simulink model "TCC"  (R2022b)
settings: configuration reference "ERT" (kept outside this file)
undefined symbols (not defined in the file): DFC, ECM, EGM, facTrqDmpGain_C, facTrqRateLim_C, FID, kiMultdtNCtrl_C, kiMultdtPosnCtrl_C, kpNCtrl_C, kpPosnCtrl_C, SpdSetAlOfsCal_C, tauTrqDmpAvrg_C, tauTrqDmpDelay_C, tiPosnHold_C, trqPMaxNCtrl_C, trqPMaxPosnCtrl_C, TrqSetAlOfsCal_C
libraries: simulink x7, DSMLib x2, MathLib x2
settings Model: Creator=M00039784  LastModifiedBy=M00039784
settings ConfigSetRef: SourceName=ERT  SourceLocation=Base Workspace

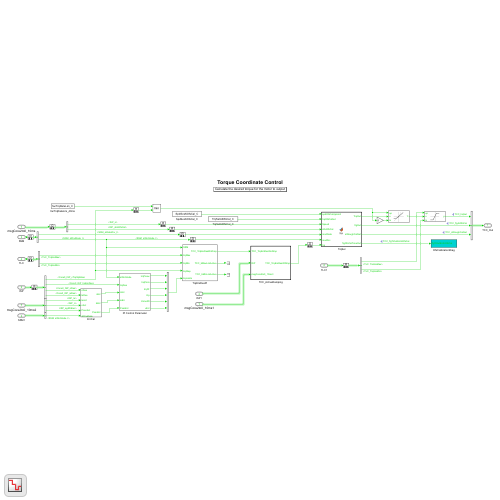
[thumbnail: Simulink's stored preview of the top-level diagram]
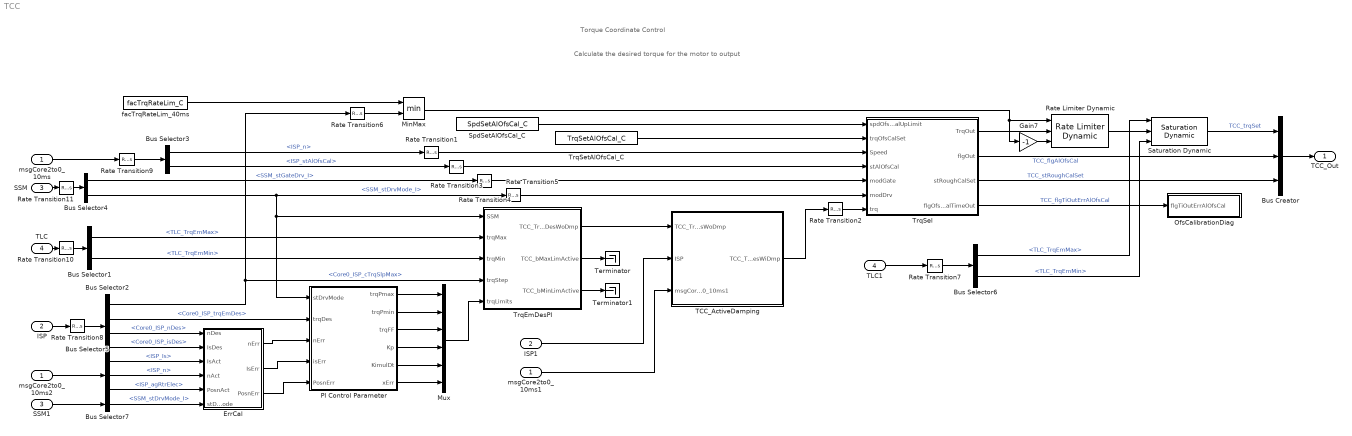
== system TCC ==
  note: Calculate the desired torque for the motor to output
  note: Torque Coordinate Control
  msgCore2to0_10ms : Inport  OutDataTypeStr=Bus: Sig10ms20ST
  ISP : Inport  Port=2  OutDataTypeStr=Bus: Core0_ISP_Out
  SSM : Inport  Port=3  OutDataTypeStr=Bus: Core0_SSM_Out
  TLC : Inport  Port=4  OutDataTypeStr=Bus: Core0_TLC_Out
  Bus Creator : BusCreator  Inputs=3
  Bus Selector1 : BusSelector  OutputSignals=TLC_TrqEmMax,TLC_TrqEmMin
  Bus Selector2 : BusSelector  OutputSignals=Core0_ISP_ComCmd.Core0_ISP_cmdx.Core0_ISP_cTrqSlpMax,Core0_ISP_ComCmd.Core0_ISP_trqx.Core0_ISP_trqEmDes,Core0_ISP_ComCmd.Core0_ISP_cmdx.Core0_ISP_nDes,Core0_ISP_ComCmd.Core0_ISP_cmdx.Core0_ISP_isDes
  Bus Selector3 : BusSelector  OutputSignals=ISP_n,ISP_stAlOfsCal
  Bus Selector4 : BusSelector  OutputSignals=SSM_stGateDrv_I,SSM_stDrvMode_I
  Bus Selector5 : BusSelector  OutputSignals=ISP_Is,ISP_n,ISP_agRtrElec
  Bus Selector6 : BusSelector  OutputSignals=TLC_TrqEmMax,TLC_TrqEmMin
  Bus Selector7 : BusSelector  OutputSignals=SSM_stDrvMode_I
  ErrCal : Subsystem
  Gain7 : Gain  Gain=-1  ParamDataTypeStr=single
  ISP1 : InportShadow  Port=2  OutDataTypeStr=Bus: Core0_ISP_Out
  MinMax : MinMax  Inputs=2
  Mux : Mux  Inputs=6
  OfsCalibrationDiag : Subsystem
  PI Control Parameter : Subsystem
  Rate Limiter Dynamic : simulink/Discontinuities/Rate Limiter Dynamic
  Rate Transition{1..3,6..7} (5 alike) : RateTransition
  Rate Transition{8..11} (4 alike) : RateTransition  OutPortSampleTime=Ts_10ms
  Rate Transition4 : RateTransition  InitialCondition=EGM.Freewheel
  Rate Transition5 : RateTransition  InitialCondition=ECM.Init
  SSM1 : InportShadow  Port=3  OutDataTypeStr=Bus: Core0_SSM_Out
  Saturation Dynamic : simulink/Discontinuities/Saturation Dynamic  OutMin=[]  OutMax=[]  OutDataTypeStr=Inherit: Same as second input  OutDataType=fixdt(1, 16)  OutScaling=2^-10  DoSatur=off
  SpdSetAlOfsCal_C : Constant  Value=SpdSetAlOfsCal_C  OutDataTypeStr=single  SampleTime=-1
  TCC_ActiveDamping : Subsystem  TreatAsAtomicUnit=on
  TLC1 : InportShadow  Port=4  OutDataTypeStr=Bus: Core0_TLC_Out
  Terminator : Terminator
  Terminator1 : Terminator
  TrqEmDesPI : Subsystem
  TrqSel : MATLAB Function
  TrqSetAlOfsCal_C : Constant  Value=TrqSetAlOfsCal_C  OutDataTypeStr=single  SampleTime=-1
  facTrqRateLim_40ms : Constant  Value=facTrqRateLim_C  OutDataTypeStr=single  SampleTime=-1
  msgCore2to0_10ms1 : InportShadow  OutDataTypeStr=Bus: Sig10ms20ST
  msgCore2to0_10ms2 : InportShadow  OutDataTypeStr=Bus: Sig10ms20ST
  TCC_Out : Outport  OutDataTypeStr=Bus: Core0_TCC_Out  VectorParamsAs1DForOutWhenUnconnected=off
  wires:
  msgCore2to0_10ms/1 -> Rate Transition9/1
  SSM1/1 -> Bus Selector7/1
  PI Control Parameter/1(trqPmax) -> Mux/1
  Rate Transition6/1 -> MinMax/2
  TCC_ActiveDamping/1(TCC_TrqEmDesWiDmp) -> Rate Transition2/1
  PI Control Parameter/4(Kp) -> Mux/4
  Bus Selector5/2 -> ErrCal/4(nAct)  "<ISP_n>"
  Bus Selector6/1 -> Saturation Dynamic/1  "<TLC_TrqEmMax>"
  Bus Selector5/1 -> ErrCal/3(IsAct)  "<ISP_Is>"
  Bus Selector1/2 -> TrqEmDesPI/3(trqMin)  "<TLC_TrqEmMin>"
  TLC/1 -> Rate Transition10/1
  TrqSel/2(flgOut) -> Bus Creator/2  "TCC_flgAlOfsCal"
  ErrCal/1(nErr) -> PI Control Parameter/3(nErr)
  ISP1/1 -> TCC_ActiveDamping/2(ISP)
  PI Control Parameter/2(trqPmin) -> Mux/2
  Bus Creator/1 -> TCC_Out/1
  SpdSetAlOfsCal_C/1 -> TrqSel/1(spdOfsCalUpLimit)
  Bus Selector5/3 -> ErrCal/5(PosnAct)  "<ISP_agRtrElec>"
  TLC1/1 -> Rate Transition7/1
  ISP/1 -> Rate Transition8/1
  Bus Selector2/4 -> ErrCal/2(IsDes)  "<Core0_ISP_isDes>"
  msgCore2to0_10ms2/1 -> Bus Selector5/1
  Rate Limiter Dynamic/1 -> Saturation Dynamic/2
  Mux/1 -> TrqEmDesPI/5(trqLimits)
  Rate Transition7/1 -> Bus Selector6/1
  msgCore2to0_10ms1/1 -> TCC_ActiveDamping/3(msgCore2to0_10ms1)
  PI Control Parameter/3(trqFF) -> Mux/3
  TrqSel/4(flgOfsCalTimeOut) -> OfsCalibrationDiag/1(flgTiOutErrAlOfsCal)  "TCC_flgTiOutErrAlOfsCal"
  TrqSetAlOfsCal_C/1 -> TrqSel/2(trqOfsCalSet)
  Bus Selector1/1 -> TrqEmDesPI/2(trqMax)  "<TLC_TrqEmMax>"
  Bus Selector2/3 -> ErrCal/1(nDes)  "<Core0_ISP_nDes>"
  TrqEmDesPI/1(TCC_TrqEmDesWoDmp) -> TCC_ActiveDamping/1(TCC_TrqEmDesWoDmp)
  TrqEmDesPI/3(TCC_bMinLimActive) -> Terminator1/1
  Bus Selector6/2 -> Saturation Dynamic/3  "<TLC_TrqEmMin>"
  TrqSel/3(stRoughCalSet) -> Bus Creator/3  "TCC_stRoughCalSet"
  PI Control Parameter/6(xErr) -> Mux/6
  Rate Transition3/1 -> TrqSel/4(stAlOfsCal)
  TrqSel/1(TrqOut) -> Rate Limiter Dynamic/2
  Rate Transition4/1 -> TrqSel/5(modGate)
  Bus Selector3/2 -> Rate Transition3/1  "<ISP_stAlOfsCal>"
  MinMax/1 -> Gain7/1, Rate Limiter Dynamic/1
  Rate Transition5/1 -> TrqSel/6(modDrv)
  Rate Transition1/1 -> TrqSel/3(Speed)
  Bus Selector2/2 -> PI Control Parameter/2(trqDes)  "<Core0_ISP_trqEmDes>"
  Rate Transition2/1 -> TrqSel/7(trq)
  ErrCal/3(PosnErr) -> PI Control Parameter/5(PosnErr)
  Bus Selector4/1 -> Rate Transition4/1  "<SSM_stGateDrv_I>"
  facTrqRateLim_40ms/1 -> MinMax/1
  Bus Selector2/1 -> TrqEmDesPI/4(trqStep), Rate Transition6/1  "<Core0_ISP_cTrqSlpMax>"
  TrqEmDesPI/2(TCC_bMaxLimActive) -> Terminator/1
  ErrCal/2(IsErr) -> PI Control Parameter/4(isErr)
  Gain7/1 -> Rate Limiter Dynamic/3
  Bus Selector3/1 -> Rate Transition1/1  "<ISP_n>"
  SSM/1 -> Rate Transition11/1
  Bus Selector7/1 -> ErrCal/6(stDrvMode)  "<SSM_stDrvMode_I>"
  PI Control Parameter/5(KimulDt) -> Mux/5
  Saturation Dynamic/1 -> Bus Creator/1  "TCC_trqSet"
  Bus Selector4/2 -> Rate Transition5/1, TrqEmDesPI/1(SSM), PI Control Parameter/1(stDrvMode)  "<SSM_stDrvMode_I>"
  Rate Transition9/1 -> Bus Selector3/1
  Rate Transition8/1 -> Bus Selector2/1
  Rate Transition10/1 -> Bus Selector1/1
  Rate Transition11/1 -> Bus Selector4/1

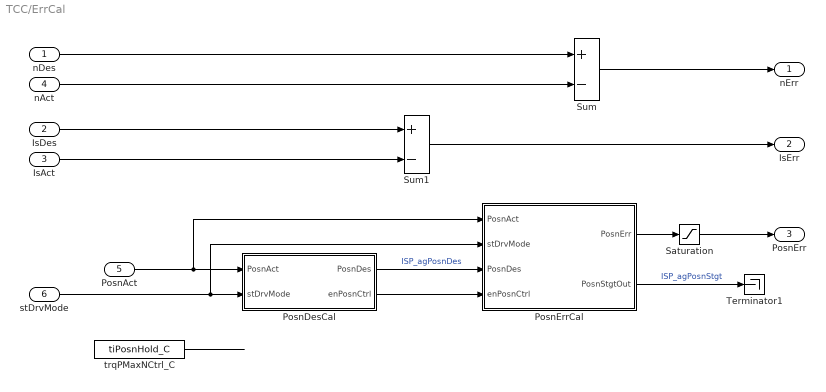
== system TCC/ErrCal ==
  nDes : Inport
  IsDes : Inport  Port=2
  IsAct : Inport  Port=3
  nAct : Inport  Port=4
  PosnAct : Inport  Port=5
  stDrvMode : Inport  Port=6
  PosnDesCal : MATLAB Function
  PosnErrCal : MATLAB Function
  Saturation : Saturate  UpperLimit=single(5000)  LowerLimit=single(-5000)
  Sum : Sum  Inputs=+-  InputSameDT=on  SaturateOnIntegerOverflow=on  OutDataTypeStr=Inherit: Same as first input
  Sum1 : Sum  Inputs=+-  InputSameDT=on  SaturateOnIntegerOverflow=on  OutDataTypeStr=Inherit: Same as first input
  Terminator1 : Terminator
  trqPMaxNCtrl_C : Constant  Value=tiPosnHold_C  OutDataTypeStr=single  SampleTime=-1
  nErr : Outport  VectorParamsAs1DForOutWhenUnconnected=off
  IsErr : Outport  Port=2  VectorParamsAs1DForOutWhenUnconnected=off
  PosnErr : Outport  Port=3  VectorParamsAs1DForOutWhenUnconnected=off
  wires:
  IsDes/1 -> Sum1/1
  Sum/1 -> nErr/1
  IsAct/1 -> Sum1/2
  Sum1/1 -> IsErr/1
  nDes/1 -> Sum/1
  nAct/1 -> Sum/2
  PosnAct/1 -> PosnErrCal/1(PosnAct), PosnDesCal/1(PosnAct)
  trqPMaxNCtrl_C/1 -> ?
  PosnDesCal/1(PosnDes) -> PosnErrCal/3(PosnDes)  "ISP_agPosnDes"
  PosnErrCal/1(PosnErr) -> Saturation/1
  stDrvMode/1 -> PosnErrCal/2(stDrvMode), PosnDesCal/2(stDrvMode)
  PosnDesCal/2(enPosnCtrl) -> PosnErrCal/4(enPosnCtrl)
  PosnErrCal/2(PosnStgtOut) -> Terminator1/1  "ISP_agPosnStgt"
  Saturation/1 -> PosnErr/1

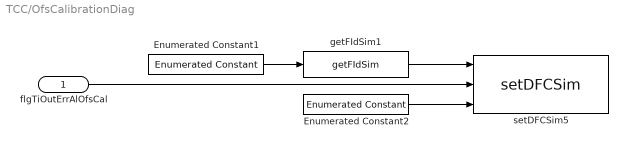
== system TCC/OfsCalibrationDiag ==
  flgTiOutErrAlOfsCal : Inport
  Enumerated Constant1 : simulink/Sources/Enumerated Constant  OutDataTypeStr=Enum: FID  Value=FID.DiagOfsCalOvrTime  SampleTime=inf
  Enumerated Constant2 : simulink/Sources/Enumerated Constant  OutDataTypeStr=Enum: DFC  Value=DFC.OfsCalOvrTime  SampleTime=inf
  getFIdSim1 : DSMLib/getFIdSim  SystemSampleTime=-1  VariantActivationTime=update diagram  Latency=0  AutoFrameSizeCalculation=off
  setDFCSim5 : DSMLib/setDFCSim  SystemSampleTime=-1  VariantActivationTime=update diagram  Latency=0  AutoFrameSizeCalculation=off
  wires:
  getFIdSim1/1 -> setDFCSim5/1
  Enumerated Constant2/1 -> setDFCSim5/3
  Enumerated Constant1/1 -> getFIdSim1/1
  flgTiOutErrAlOfsCal/1 -> setDFCSim5/2

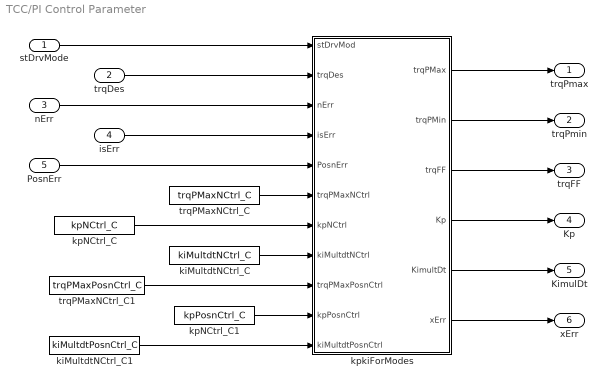
== system TCC/PI Control Parameter ==
  stDrvMode : Inport
  trqDes : Inport  Port=2
  nErr : Inport  Port=3
  isErr : Inport  Port=4
  PosnErr : Inport  Port=5
  kiMultdtNCtrl_C : Constant  Value=kiMultdtNCtrl_C  OutDataTypeStr=single  SampleTime=-1
  kiMultdtNCtrl_C1 : Constant  Value=kiMultdtPosnCtrl_C  OutDataTypeStr=single  SampleTime=-1
  kpNCtrl_C : Constant  Value=kpNCtrl_C  OutDataTypeStr=single  SampleTime=-1
  kpNCtrl_C1 : Constant  Value=kpPosnCtrl_C  OutDataTypeStr=single  SampleTime=-1
  kpkiForModes : MATLAB Function
  trqPMaxNCtrl_C : Constant  Value=trqPMaxNCtrl_C  OutDataTypeStr=single  SampleTime=-1
  trqPMaxNCtrl_C1 : Constant  Value=trqPMaxPosnCtrl_C  OutDataTypeStr=single  SampleTime=-1
  trqPmax : Outport  VectorParamsAs1DForOutWhenUnconnected=off
  trqPmin : Outport  Port=2  VectorParamsAs1DForOutWhenUnconnected=off
  trqFF : Outport  Port=3  VectorParamsAs1DForOutWhenUnconnected=off
  Kp : Outport  Port=4  VectorParamsAs1DForOutWhenUnconnected=off
  KimulDt : Outport  Port=5  VectorParamsAs1DForOutWhenUnconnected=off
  xErr : Outport  Port=6  VectorParamsAs1DForOutWhenUnconnected=off
  wires:
  trqDes/1 -> kpkiForModes/2(trqDes)
  kpNCtrl_C/1 -> kpkiForModes/7(kpNCtrl)
  kpkiForModes/5(KimultDt) -> KimulDt/1
  kpkiForModes/3(trqFF) -> trqFF/1
  kpkiForModes/6(xErr) -> xErr/1
  trqPMaxNCtrl_C/1 -> kpkiForModes/6(trqPMaxNCtrl)
  kiMultdtNCtrl_C/1 -> kpkiForModes/8(kiMultdtNCtrl)
  kpkiForModes/1(trqPMax) -> trqPmax/1
  kpkiForModes/4(Kp) -> Kp/1
  kpkiForModes/2(trqPMin) -> trqPmin/1
  isErr/1 -> kpkiForModes/4(isErr)
  nErr/1 -> kpkiForModes/3(nErr)
  PosnErr/1 -> kpkiForModes/5(PosnErr)
  stDrvMode/1 -> kpkiForModes/1(stDrvMod)
  trqPMaxNCtrl_C1/1 -> kpkiForModes/9(trqPMaxPosnCtrl)
  kpNCtrl_C1/1 -> kpkiForModes/10(kpPosnCtrl)
  kiMultdtNCtrl_C1/1 -> kpkiForModes/11(kiMultdtPosnCtrl)

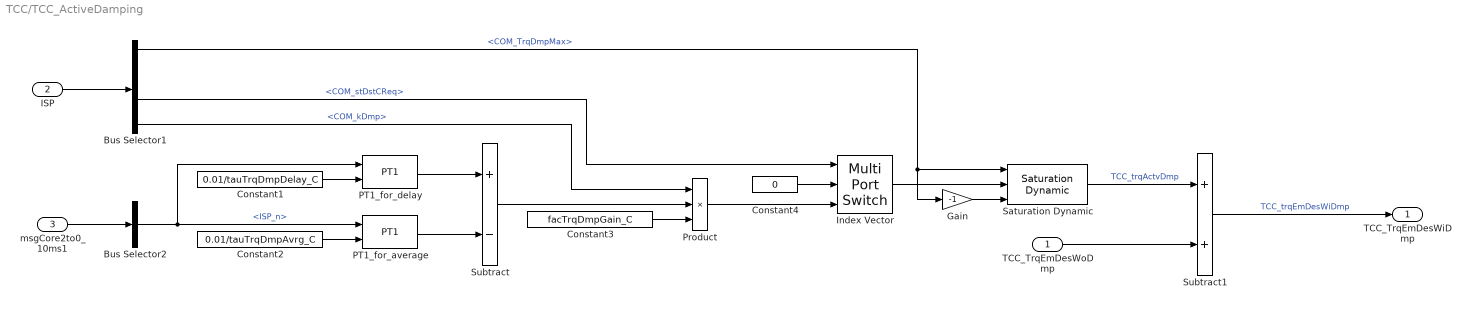
== system TCC/TCC_ActiveDamping ==
  TCC_TrqEmDesWoDmp : Inport
  ISP : Inport  Port=2
  msgCore2to0_10ms1 : Inport  Port=3
  Bus Selector1 : BusSelector  OutputSignals=Core0_ISP_ComCmd.Com_Msg06.COM_TrqDmpMax,Core0_ISP_ComCmd.Com_Msg06.COM_TrqDmpLim,Core0_ISP_ComCmd.Com_Msg06.COM_stDstCReq,Core0_ISP_ComCmd.Com_Msg06.COM_kDmp
  Bus Selector2 : BusSelector  OutputSignals=ISP_n
  Constant1 : Constant  Value=0.01/tauTrqDmpDelay_C  OutDataTypeStr=single
  Constant2 : Constant  Value=0.01/tauTrqDmpAvrg_C  OutDataTypeStr=single
  Constant3 : Constant  Value=facTrqDmpGain_C  OutDataTypeStr=single
  Constant4 : Constant  Value=0  OutDataTypeStr=single
  Gain : Gain  Gain=-1
  Index Vector : MultiPortSwitch  DataPortOrder=Zero-based contiguous  Inputs=2  zeroidx=on  OutDataTypeStr=single  SaturateOnIntegerOverflow=off  InputSameDT=off
  PT1_for_average : MathLib/PT1  SystemSampleTime=-1  VariantActivationTime=update diagram  Latency=0  AutoFrameSizeCalculation=off
  PT1_for_delay : MathLib/PT1  SystemSampleTime=-1  VariantActivationTime=update diagram  Latency=0  AutoFrameSizeCalculation=off
  Product : Product  Inputs=3
  Saturation Dynamic : simulink/Discontinuities/Saturation Dynamic  OutMin=[]  OutMax=[]  OutDataTypeStr=Inherit: Same as second input  OutDataType=fixdt(1, 16)  OutScaling=2^-10  DoSatur=off
  Subtract : Sum  Inputs=+-
  Subtract1 : Sum
  TCC_TrqEmDesWiDmp : Outport  VectorParamsAs1DForOutWhenUnconnected=off
  wires:
  msgCore2to0_10ms1/1 -> Bus Selector2/1
  Constant2/1 -> PT1_for_average/2
  PT1_for_average/1 -> Subtract/2
  Constant1/1 -> PT1_for_delay/2
  Bus Selector2/1 -> PT1_for_average/1, PT1_for_delay/1  "<ISP_n>"
  PT1_for_delay/1 -> Subtract/1
  Subtract/1 -> Product/2
  Constant3/1 -> Product/3
  ISP/1 -> Bus Selector1/1
  Product/1 -> Index Vector/3
  Constant4/1 -> Index Vector/2
  Bus Selector1/4 -> Product/1  "<COM_kDmp>"
  Bus Selector1/3 -> Index Vector/1  "<COM_stDstCReq>"
  Index Vector/1 -> Saturation Dynamic/2
  Bus Selector1/1 -> Gain/1, Saturation Dynamic/1  "<COM_TrqDmpMax>"
  TCC_TrqEmDesWoDmp/1 -> Subtract1/2
  Subtract1/1 -> TCC_TrqEmDesWiDmp/1  "TCC_trqEmDesWiDmp"
  Saturation Dynamic/1 -> Subtract1/1  "TCC_trqActvDmp"
  Gain/1 -> Saturation Dynamic/3

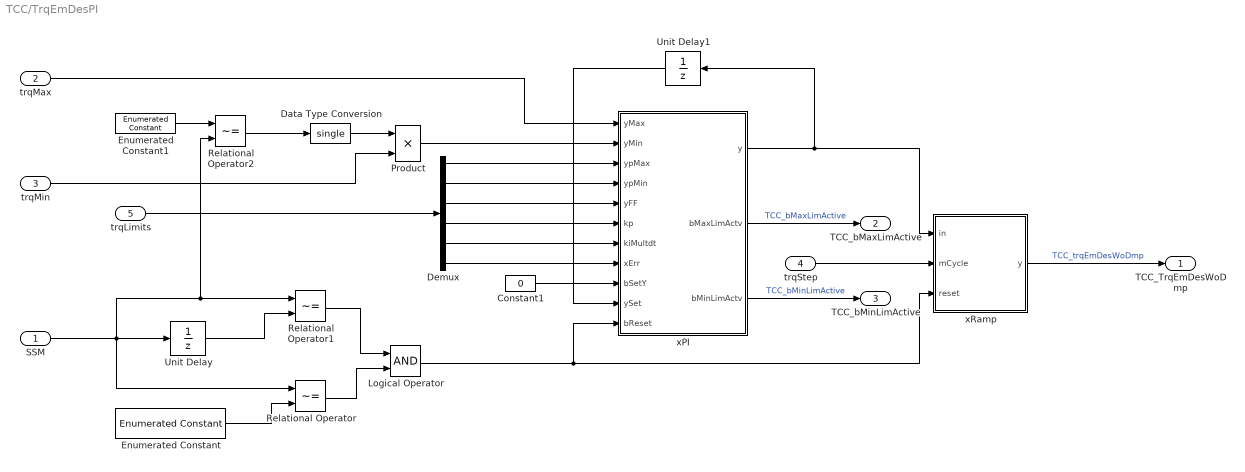
== system TCC/TrqEmDesPI ==
  SSM : Inport
  trqMax : Inport  Port=2
  trqMin : Inport  Port=3
  trqStep : Inport  Port=4
  trqLimits : Inport  Port=5
  Constant1 : Constant  Value=0  OutDataTypeStr=boolean
  Data Type Conversion : DataTypeConversion  OutDataTypeStr=single  SaturateOnIntegerOverflow=off  RndMeth=Floor
  Demux : Demux  Outputs=6
  Enumerated Constant : simulink/Sources/Enumerated Constant  OutDataTypeStr=Enum: ECM  Value=ECM.Standby  SampleTime=inf
  Enumerated Constant1 : simulink/Sources/Enumerated Constant  OutDataTypeStr=Enum: ECM  Value=ECM.IsCtrl  SampleTime=inf
  Logical Operator : Logic  AllPortsSameDT=off  OutDataTypeStr=boolean
  Product : Product  Inputs=**  InputSameDT=on  RndMeth=Zero  SaturateOnIntegerOverflow=on  OutDataTypeStr=Inherit: Same as first input
  Relational Operator : RelationalOperator  Operator=~=  OutDataTypeStr=boolean  RndMeth=Simplest  InputSameDT=off
  Relational Operator1 : RelationalOperator  Operator=~=  OutDataTypeStr=boolean  RndMeth=Simplest  InputSameDT=off
  Relational Operator2 : RelationalOperator  Operator=~=  OutDataTypeStr=boolean  RndMeth=Simplest  InputSameDT=off
  Unit Delay : UnitDelay  InitialCondition=ECM.Init  SampleTime=-1  HasFrameUpgradeWarning=on
  Unit Delay1 : UnitDelay  SampleTime=-1  HasFrameUpgradeWarning=on
  xPI : MATLAB Function  TreatAsAtomicUnit=on
  xRamp : MATLAB Function  TreatAsAtomicUnit=on
  TCC_TrqEmDesWoDmp : Outport  VectorParamsAs1DForOutWhenUnconnected=off
  TCC_bMaxLimActive : Outport  Port=2  VectorParamsAs1DForOutWhenUnconnected=off
  TCC_bMinLimActive : Outport  Port=3  VectorParamsAs1DForOutWhenUnconnected=off
  wires:
  SSM/1 -> Relational Operator/1, Unit Delay/1, Relational Operator2/2, Relational Operator1/1
  Unit Delay/1 -> Relational Operator1/2
  Enumerated Constant/1 -> Relational Operator/2
  Relational Operator/1 -> Logical Operator/2
  Relational Operator1/1 -> Logical Operator/1
  trqMax/1 -> xPI/1(yMax)
  Constant1/1 -> xPI/9(bSetY)
  Logical Operator/1 -> xRamp/3(reset), xPI/11(bReset)
  Relational Operator2/1 -> Data Type Conversion/1
  Product/1 -> xPI/2(yMin)
  trqMin/1 -> Product/2
  Enumerated Constant1/1 -> Relational Operator2/1
  Demux/6 -> xPI/8(xErr)
  Demux/5 -> xPI/7(kiMultdt)
  Demux/4 -> xPI/6(kp)
  Demux/3 -> xPI/5(yFF)
  Demux/1 -> xPI/3(ypMax)
  Demux/2 -> xPI/4(ypMin)
  Data Type Conversion/1 -> Product/1
  Unit Delay1/1 -> xPI/10(ySet)
  trqStep/1 -> xRamp/2(mCycle)
  xRamp/1(y) -> TCC_TrqEmDesWoDmp/1  "TCC_trqEmDesWoDmp"
  xPI/3(bMinLimActv) -> TCC_bMinLimActive/1  "TCC_bMinLimActive"
  xPI/2(bMaxLimActv) -> TCC_bMaxLimActive/1  "TCC_bMaxLimActive"
  xPI/1(y) -> Unit Delay1/1, xRamp/1(in)
  trqLimits/1 -> Demux/1

== matlab function TCC/TrqSel ==
  data: spdOfsCalUpLimit input; trqOfsCalSet input; Speed input; stAlOfsCal input; modGate input; modDrv input; trq input; TrqOut output; flgOut output; stRoughCalSet output; flgOfsCalTimeOut output
function [TrqOut,flgOut,stRoughCalSet,flgOfsCalTimeOut]   = fcn(spdOfsCalUpLimit,trqOfsCalSet,Speed,stAlOfsCal,modGate,modDrv,trq)
%
persistent flgAlOfsCal;
persistent tiAlOfsCal;
persistent flgOfsCalTimeOutTmp;

if isempty(flgAlOfsCal)
    flgAlOfsCal = false;
    tiAlOfsCal = uint16(0);
    flgOfsCalTimeOutTmp = false;
end

if (modGate==EGM.PWMRun)
    if (modDrv==ECM.TrqCtrl)||(modDrv==ECM.nCtrl)||(modDrv==ECM.IsCtrl)||(modDrv==ECM.PosnCtrl)
        TrqOut = trq;
        stRoughCalSet = uint8(0);
    elseif (modDrv==ECM.alOfsCal)
        tiAlOfsCal = tiAlOfsCal + uint16(1);
        %step1:find rough 0 position
        if tiAlOfsCal<uint16(500)  %0.5s
            TrqOut = single(0);
            stRoughCalSet = uint8(1);
        elseif tiAlOfsCal<uint16(1000)  %1s
            TrqOut = single(0);
            stRoughCalSet = uint8(2);
        elseif tiAlOfsCal<uint16(1500)  %1.5s
            TrqOut = single(0);
            stRoughCalSet = uint8(3); 
        elseif tiAlOfsCal<uint16(2000)  %2s
            TrqOut = single(0);
            stRoughCalSet = uint8(4);   
        %step2:find accurate 0 position
        elseif tiAlOfsCal<uint16(5000)  %2~5s
            stRoughCalSet = uint8(5);
            if  (Speed<spdOfsCalUpLimit)&&(flgAlOfsCal==false)
                TrqOut = trqOfsCalSet;
            else 
                flgAlOfsCal = true;
                if (Speed>single(200))&&(stAlOfsCal~=uint8(0))
                    TrqOut = single(0); %-trqOfsCalSet; change to 0 because Vdc overvoltage
                else
                    TrqOut = single(0);
                end
            end
        else
            TrqOut = single(0);
            stRoughCalSet = uint8(0);
            tiAlOfsCal = uint16(6000);
            flgAlOfsCal = false;
            flgOfsCalTimeOutTmp = true;
        end
    else
        TrqOut = single(0);
        stRoughCalSet = uint8(0);
        flgAlOfsCal = false;
    end
else
    TrqOut = single(0);
    stRoughCalSet = uint8(0);
    flgAlOfsCal = false;
    tiAlOfsCal = uint16(0);
end

flgOut = flgAlOfsCal;
flgOfsCalTimeOut = flgOfsCalTimeOutTmp;

== matlab function TCC/ErrCal/PosnDesCal ==
  data: PosnAct input; stDrvMode input; PosnDes output; enPosnCtrl output
function [PosnDes,enPosnCtrl] = fcn(PosnAct,stDrvMode)
%
persistent stDrvModeLast;
persistent TempPosnAct;
persistent TempEnPosnCtrl;

if isempty(stDrvModeLast)
    stDrvModeLast = ECM.PreInit;
    TempPosnAct = single(0.0);
    TempEnPosnCtrl = false;
end

if (stDrvMode==ECM.PosnCtrl)&&(stDrvModeLast==ECM.TrqCtrl)
    TempPosnAct = PosnAct;
    TempEnPosnCtrl = true;
end

if stDrvMode~=ECM.PosnCtrl
    TempEnPosnCtrl = false;
end

stDrvModeLast = stDrvMode;
PosnDes = TempPosnAct;
enPosnCtrl = TempEnPosnCtrl;

== matlab function TCC/ErrCal/PosnErrCal ==
  data: PosnAct input; stDrvMode input; PosnDes input; PosnErr output; enPosnCtrl input; PosnStgtOut output
function [PosnErr,PosnStgtOut]    = fcn(PosnAct,stDrvMode,PosnDes,enPosnCtrl)
%
%100rpm,4Pair poles: T=0.15s
persistent TempPosnActLast;
persistent PosnStgt;  %Posntion straightening

if isempty(TempPosnActLast)
    TempPosnActLast = single(0);
    PosnStgt = single(0);
end

dPosn = PosnAct - TempPosnActLast;
TempPosnActLast = PosnAct;

%for 0.1m vechile move
%for tire with 0.5m radius, motor with 4poles
%45deg will turn
if abs(dPosn)<single(16383)
    dPosnRctf = dPosn;%Position rectify
elseif abs(dPosn)>single(49152)
    if dPosn>single(0)
        dPosnRctf = single(-65535) + dPosn;
    else
        dPosnRctf = single(65535) + dPosn;
    end
else
    dPosnRctf = single(0);
end
    
if (stDrvMode==ECM.PosnCtrl)&&enPosnCtrl
    PosnStgt = PosnStgt + dPosnRctf;
    PosnErr = PosnDes - PosnStgt;
else
    PosnStgt = PosnAct;
    PosnErr = single(0);
end

PosnStgtOut = PosnStgt;

== matlab function TCC/PI Control Parameter/kpkiForModes ==
  data: stDrvMod input; trqDes input; nErr input; isErr input; PosnErr input; trqPMax output; trqPMin output; trqFF output; Kp output; KimultDt output; xErr output; trqPMaxNCtrl input; kpNCtrl input; kiMultdtNCtrl input; trqPMaxPosnCtrl input; kpPosnCtrl input; kiMultdtPosnCtrl input
function [trqPMax,trqPMin,trqFF,Kp,KimultDt,xErr]...
         = fcn(stDrvMod,trqDes,nErr,isErr,PosnErr,trqPMaxNCtrl,kpNCtrl,kiMultdtNCtrl,trqPMaxPosnCtrl,kpPosnCtrl,kiMultdtPosnCtrl)
%
switch stDrvMod
    case ECM.TrqCtrl
        trqPMax = single(0);
        trqPMin = single(0);
        trqFF = trqDes;
        Kp = single(0);
        KimultDt = single(0);
        xErr = single(0);
    case ECM.nCtrl
        trqPMax = trqPMaxNCtrl; %trqPMaxNCtrl_C
        trqPMin = -trqPMaxNCtrl; %-trqPMaxNCtrl_C
        trqFF = single(0);
        Kp = kpNCtrl; %kpNCtrl_C
        KimultDt = kiMultdtNCtrl; %kiMultdtNCtrl_C
        xErr = nErr;
    case ECM.PosnCtrl
        trqPMax = trqPMaxPosnCtrl;
        trqPMin = -trqPMaxPosnCtrl; 
        trqFF = single(0);
        Kp = kpPosnCtrl;
        KimultDt = kiMultdtPosnCtrl;
        xErr = PosnErr;
    case ECM.IsCtrl
        trqPMax = single(0);
        trqPMin = single(0);
        trqFF = trqDes;
        Kp = single(0);
        KimultDt = single(0);
        xErr = isErr;
    otherwise
        trqPMax = single(0);
        trqPMin = single(0);
        trqFF = single(0);
        Kp = single(0);
        KimultDt = single(0);
        xErr = single(0);
end

== matlab function TCC/TrqEmDesPI/xPI ==
  data: yMax input; yMin input; ypMax input; y output; ypMin input; yFF input; kp input; kiMultdt input; xErr input; bSetY input; ySet input; bReset input; bMaxLimActv output; bMinLimActv output
function [y,bMaxLimActv,bMinLimActv] = xPI(yMax,yMin,ypMax,ypMin,yFF,kp,kiMultdt,xErr,bSetY,ySet,bReset)
persistent yi;

if isempty(yi)
    yi = single(0);
end

if bReset
    bMaxLimActv = false;
    bMinLimActv = false;
    yi = ySet;
    y = ySet;
else
     yiAdd = kiMultdt*xErr;
     yp = max(min(kp*xErr, ypMax),ypMin);	
     ypSumyFF = yp + yFF;
     if bSetY					% set output: y = ySet	
     	yi = ySet - ypSumyFF - yiAdd;
     end
     
     yiNew = yiAdd + yi;
     yUnlim = yiNew + ypSumyFF;
 
     if (yUnlim >= yMax) 		% controller limited by yMax
     	bMaxLimActv = true;
        bMinLimActv = false;
     	y = yMax;
     	yi = max((yMax - ypSumyFF), 0);
     elseif(yUnlim <= yMin)     % controller limited by yMin
        bMaxLimActv = false;
        bMinLimActv = true;
        y = yMin;
        yi = min((yMin - ypSumyFF), 0);
     else                       % controller not limited
        bMaxLimActv = false;
        bMinLimActv = false;
        y = (yUnlim);
        yi = (yiNew);
     end
end

== matlab function TCC/TrqEmDesPI/xRamp ==
  data: in input; y output; mCycle input; reset input
function y = xRamp(in,mCycle,reset)
persistent out;
if isempty(out)
    out = single(0);
end

if (reset) 
	out = in;
else                        % Reset condition ramp off
	dy = in - out;			% determine the maximum possible jump
	mCycleTmp = mCycle;		% only one push operator is required
	dy = min(mCycleTmp, dy);	% Limit the jump by increasing the slope
	dy = max(-mCycleTmp,dy);    % Limit the jump by downward slope
	out = (out + dy);           %  Jump to output.
end

y=out;
end
